simulink model "nichtlinearesModell"  (R2016b)
settings: Solver=VariableStepAuto  StartTime=0.0  StopTime=15  RelTol=1e-3
values from neighbouring files (symbols this model uses):
  K1 = 1    [StartSim.m]
  K2 = 1    [StartSim.m]
  L_0 = 0.2    [StartSim.m]
  phi_0 = 0    [StartSim.m]
  r1 = 0.05    [StartSim.m]
  r2 = 0.05    [StartSim.m]
  T1 = 0.05    [StartSim.m]
  T2 = 0.05    [StartSim.m]
  ue1 = 6    [StartSim.m]
  ue2 = 3    [StartSim.m]
  x_0 = 0    [StartSim.m]
undefined symbols (not defined in the file or in its folder): t01, t02, t1, t2, u1, u2
libraries: simulink_extras x2
settings Model: Creator=Patrick  LastModifiedBy=Patrick

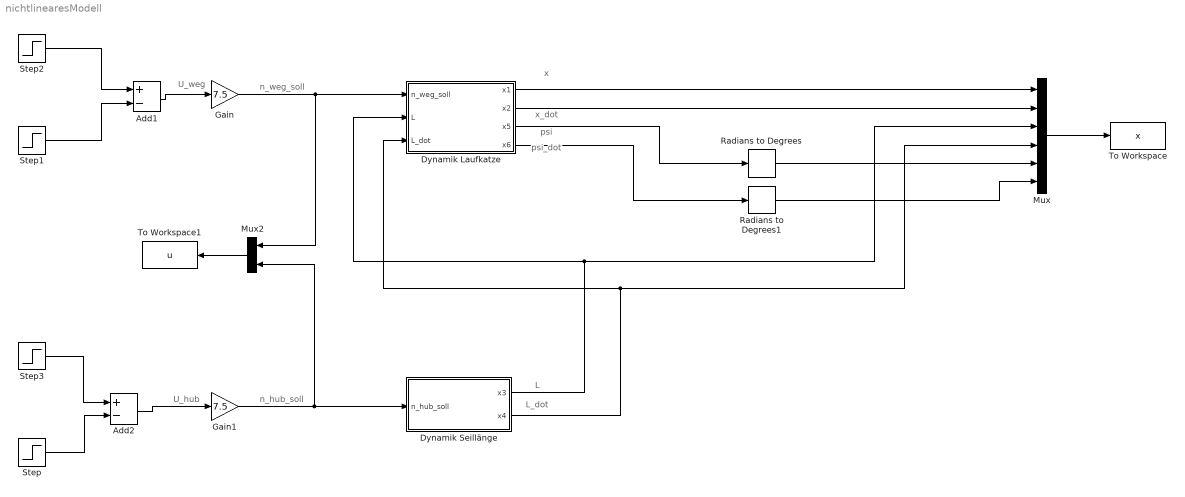
== system nichtlinearesModell ==
  note: n_hub_soll
  note: U_hub
  note: U_weg
  note: n_weg_soll
  note: L
  note: L_dot
  note: x
  note: x_dot
  note: psi
  note: psi_dot
  Add1 : Sum  Inputs=+-
  Add2 : Sum  Inputs=+-
  Dynamik Laufkatze : Subsystem
  Dynamik Seillänge : Subsystem
  Gain : Gain  Gain=7.5
  Gain1 : Gain  Gain=7.5
  Mux : Mux  Inputs=6
  Mux2 : Mux  Inputs=2
  Radians to Degrees : simulink_extras/Transformations/Radians to Degrees
  Radians to Degrees1 : simulink_extras/Transformations/Radians to Degrees
  Step : Step  Time=t2  After=u2  SampleTime=0
  Step1 : Step  Time=t1  After=u1  SampleTime=0
  Step2 : Step  Time=t01  After=u1  SampleTime=0
  Step3 : Step  Time=t02  After=u2  SampleTime=0
  To Workspace : ToWorkspace  VariableName=x  SampleTime=-1
  To Workspace1 : ToWorkspace  VariableName=u  SampleTime=-1
  wires:
  Dynamik Laufkatze/1(x1) -> Mux/1
  Dynamik Laufkatze/2(x2) -> Mux/2
  Dynamik Laufkatze/3(x5) -> Radians to Degrees/1
  Dynamik Laufkatze/4(x6) -> Radians to Degrees1/1
  Mux/1 -> To Workspace/1
  Add1/1 -> Gain/1
  Step2/1 -> Add1/1
  Add2/1 -> Gain1/1
  Gain1/1 -> Dynamik Seillänge/1(n_hub_soll), Mux2/2
  Step3/1 -> Add2/1
  Gain/1 -> Mux2/1, Dynamik Laufkatze/1(n_weg_soll)
  Dynamik Seillänge/1(x3) -> Dynamik Laufkatze/2(L), Mux/3
  Step/1 -> Add2/2
  Step1/1 -> Add1/2
  Dynamik Seillänge/2(x4) -> Dynamik Laufkatze/3(L_dot), Mux/4
  Radians to Degrees/1 -> Mux/5
  Radians to Degrees1/1 -> Mux/6
  Mux2/1 -> To Workspace1/1

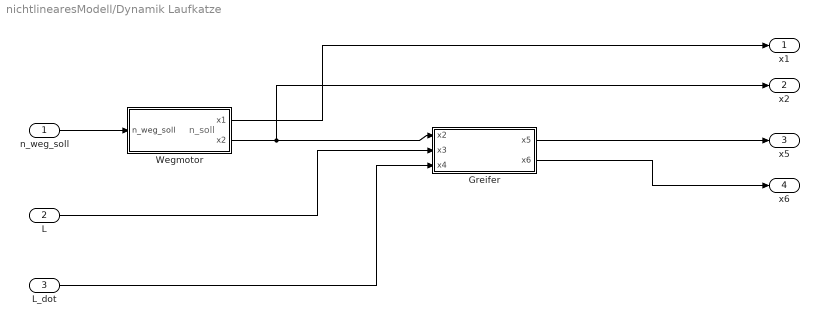
== system nichtlinearesModell/Dynamik Laufkatze ==
  note: n_soll
  n_weg_soll : Inport
  L : Inport  Port=2
  L_dot : Inport  Port=3
  Greifer : Subsystem
  Wegmotor : Subsystem
  x1 : Outport
  x2 : Outport  Port=2
  x5 : Outport  Port=3
  x6 : Outport  Port=4
  wires:
  n_weg_soll/1 -> Wegmotor/1(n_weg_soll)
  Wegmotor/1(x1) -> x1/1
  Wegmotor/2(x2) -> x2/1, Greifer/1(x2)
  Greifer/1(x5) -> x5/1
  Greifer/2(x6) -> x6/1
  L/1 -> Greifer/2(x3)
  L_dot/1 -> Greifer/3(x4)

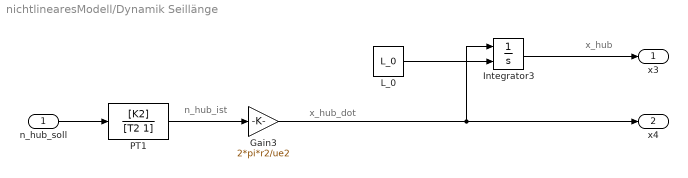
== system nichtlinearesModell/Dynamik Seillänge ==
  note: n_hub_ist
  note: x_hub_dot
  note: x_hub
  n_hub_soll : Inport
  Gain3 : Gain  Gain=2*pi*r2/ue2
  Integrator3 : Integrator  InitialConditionSource=external
  L_0 : Constant  Value=L_0
  PT1 : TransferFcn  Numerator=[K2]  Denominator=[T2 1]
  x3 : Outport
  x4 : Outport  Port=2
  wires:
  n_hub_soll/1 -> PT1/1
  PT1/1 -> Gain3/1
  Integrator3/1 -> x3/1
  L_0/1 -> Integrator3/2
  Gain3/1 -> Integrator3/1, x4/1

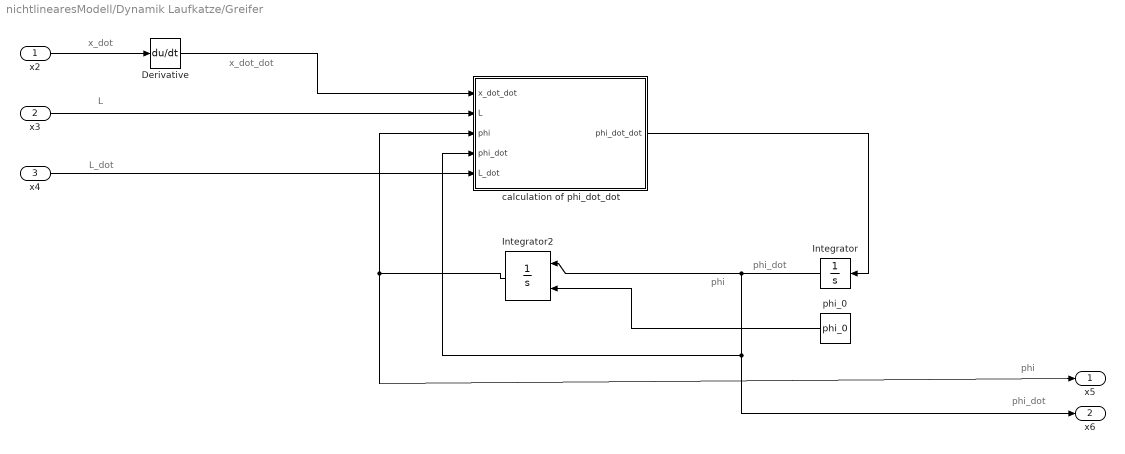
== system nichtlinearesModell/Dynamik Laufkatze/Greifer ==
  note: phi
  note: phi
  note: x_dot
  note: L
  note: phi_dot
  note: phi_dot
  note: x_dot_dot
  note: L_dot
  x2 : Inport
  x3 : Inport  Port=2
  x4 : Inport  Port=3
  Derivative : Derivative
  Integrator : Integrator
  Integrator2 : Integrator  InitialConditionSource=external
  calculation of phi_dot_dot : MATLAB Function  TreatAsAtomicUnit=on
  phi_0 : Constant  Value=phi_0
  x5 : Outport
  x6 : Outport  Port=2
  wires:
  Derivative/1 -> calculation of phi_dot_dot/1(x_dot_dot)
  x2/1 -> Derivative/1
  Integrator/1 -> x6/1, calculation of phi_dot_dot/4(phi_dot), Integrator2/1
  x3/1 -> calculation of phi_dot_dot/2(L)
  calculation of phi_dot_dot/1(phi_dot_dot) -> Integrator/1
  Integrator2/1 -> x5/1, calculation of phi_dot_dot/3(phi)
  x4/1 -> calculation of phi_dot_dot/5(L_dot)
  phi_0/1 -> Integrator2/2

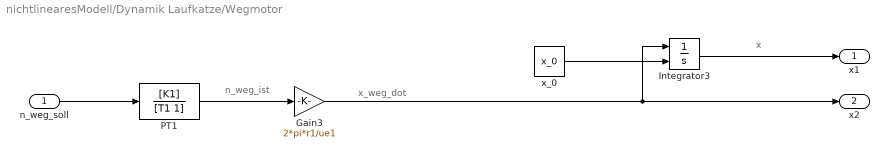
== system nichtlinearesModell/Dynamik Laufkatze/Wegmotor ==
  note: n_weg_ist
  note: x
  note: x_weg_dot
  n_weg_soll : Inport
  Gain3 : Gain  Gain=2*pi*r1/ue1
  Integrator3 : Integrator  InitialConditionSource=external
  PT1 : TransferFcn  Numerator=[K1]  Denominator=[T1 1]
  x_0 : Constant  Value=x_0
  x1 : Outport
  x2 : Outport  Port=2
  wires:
  x_0/1 -> Integrator3/2
  n_weg_soll/1 -> PT1/1
  PT1/1 -> Gain3/1
  Integrator3/1 -> x1/1
  Gain3/1 -> Integrator3/1, x2/1

== matlab function nichtlinearesModell/Dynamik Laufkatze/Greifer/calculation of phi_dot_dot ==
  data: x_dot_dot input; phi_dot_dot output; L input; phi input; phi_dot input; L_dot input
function phi_dot_dot = fcn(x_dot_dot,L,phi,phi_dot,L_dot)

phi_dot_dot = -(cos(phi)/L)*x_dot_dot-9.81/L*sin(phi)-2*L_dot*phi_dot;
